simulink model "DC_Motor_PID_Control"  (R2017b)
settings: Solver=FixedStepAuto  StartTime=0.0  StopTime=20  FixedStep=Dt  RelTol=1e-3
values from neighbouring files (symbols this model uses):
  den = [1 3 3 1]    [Run_DC_Motor_PID_Control.m]
  Kd = 8*3.6/8    (= 3.6)    [Run_DC_Motor_PID_Control.m]
  Ki = 2*8/3.6    (= 4.44444444444)    [Run_DC_Motor_PID_Control.m]
  Kp = 4.8    [Run_DC_Motor_PID_Control.m]
  num = [1]    [Run_DC_Motor_PID_Control.m]
libraries: simulink_extras x1
settings Model: Creator=Daslab  LastModifiedBy=Daslab

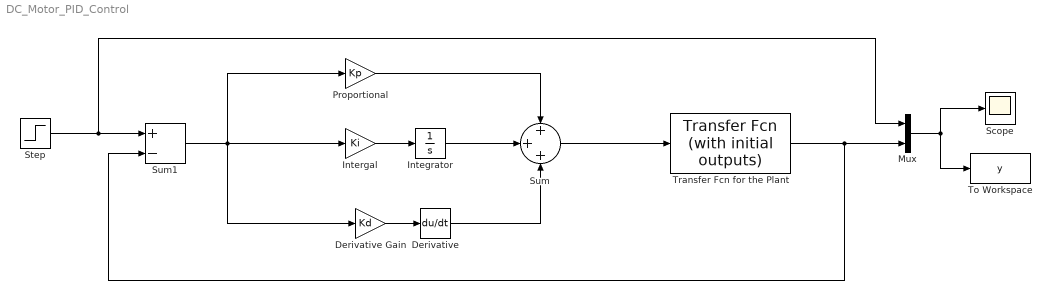
== system DC_Motor_PID_Control ==
  Derivative : Derivative  CoefficientInTFapproximation=1
  Derivative Gain : Gain  Gain=Kd
  Integrator : Integrator
  "Intergal " : Gain  Gain=Ki
  Mux : Mux  Inputs=2
  "Proportional " : Gain  Gain=Kp
  Scope : Scope
  Step : Step  Time=0  SampleTime=0
  Sum : Sum  Inputs=+++
  Sum1 : Sum  Inputs=+-
  To Workspace : ToWorkspace  VariableName=y  SaveFormat=Timeseries  SampleTime=-1
  Transfer Fcn for the Plant : simulink_extras/Additional Linear/Transfer Fcn (with initial outputs)  N=num  D=den  Y0=0  U0=0
  wires:
  "Intergal "/1 -> Integrator/1
  Derivative Gain/1 -> Derivative/1
  "Proportional "/1 -> Sum/1
  Integrator/1 -> Sum/2
  Derivative/1 -> Sum/3
  Sum/1 -> Transfer Fcn for the Plant/1
  Sum1/1 -> Derivative Gain/1, "Proportional "/1, "Intergal "/1
  Step/1 -> Mux/1, Sum1/1
  Transfer Fcn for the Plant/1 -> Mux/2, Sum1/2
  Mux/1 -> Scope/1, To Workspace/1
